simulink model "satelite01"  (Simulink 8.5)
settings: Solver=ode4  StartTime=0.0  StopTime=tfin  FixedStep=1/80
values from neighbouring files (symbols this model uses):
  A = [0 0 0.25 0.75 0 0;         0 0 0 0 2.52632 0;         0.75 0 0 0 0 0;         1 0 0 0 0 1;     0 1 0 0 0 0;     0 0 1 -1 0 0]    [Acoplado.m]    (also in insat03.m)
  B = [-0.25 0 0;     0 -0.842105 0;     0 0 0.75;     0 0 0;     0 0 0;     0 0 0]    [Acoplado.m]    (also in insat03.m = [-0.25 0 0;0 -0.842105 0;0 0 0.75)
  C = eye(6,6)    [Acoplado.m]    (also in insat03.m)
  D = zeros(6,3)    [Acoplado.m]    (also in insat03.m)
  ic = [0 0 0 0 0 0]    [Acoplado.m]    (also in insat03.m)
undefined symbols (not defined in the file or in its folder): K
libraries: simulink x1
settings Model: Creator=Vargas  LastModifiedBy=Admin
settings DataIOCC: SignalLoggingName=sigsOut
settings OptimizationCC: BlockReduction=off  BooleanDataType=off  InitFltsAndDblsToZero=on
settings DebuggingCC: SaveWithParameterizedLinksMsg=none  SignalResolutionControl=TryResolveAllWithWarning  MultiTaskDSMMsg=warning  MultiTaskCondExecSysMsg=none  FcnCallInpInsideContextMsg=UseLocalSettings  StrictBusMsg=None
settings HardwareCC: TargetUnknown=on

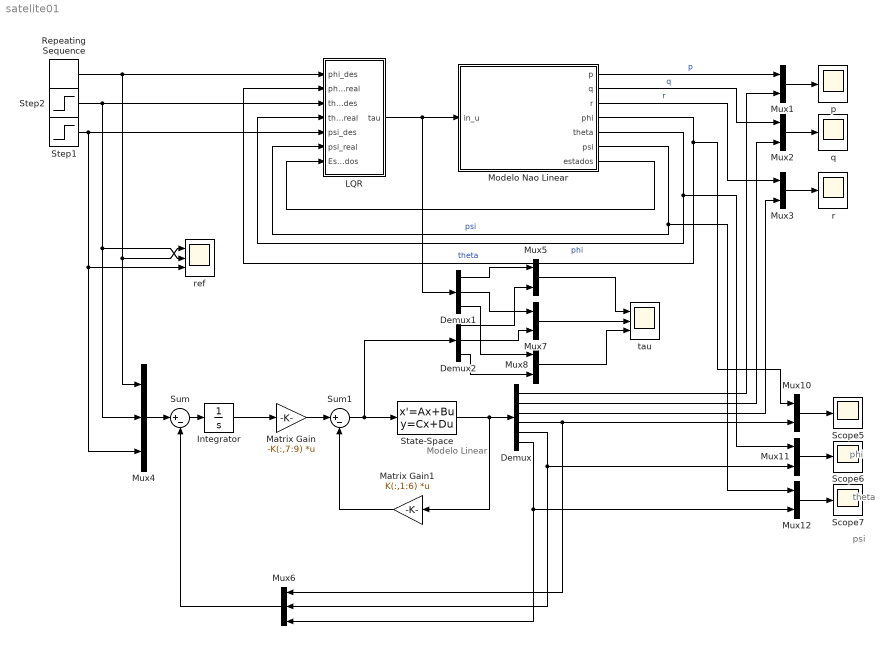
== system satelite01 ==
  note: phi
  note: theta
  note: psi
  note: Modelo Linear
  Demux : Demux  Outputs=6
  Demux1 : Demux  Outputs=3
  Demux2 : Demux  Outputs=3
  Integrator : Integrator
  LQR : Subsystem
  Matrix Gain : Gain  Gain=-K(:,7:9)  Multiplication=Matrix(K*u)  SaturateOnIntegerOverflow=on  OutDataTypeStr=Inherit: Same as input  ParamDataTypeStr=Inherit: Same as input
  Matrix Gain1 : Gain  Gain=K(:,1:6)  Multiplication=Matrix(K*u)  SaturateOnIntegerOverflow=on  OutDataTypeStr=Inherit: Same as input  ParamDataTypeStr=Inherit: Same as input
  Modelo Nao Linear : Subsystem
      mask Display: image(imread('Satelite3DOF_02.png'))
  Mux{1..3,5,7..8,10..12} (9 alike) : Mux  Inputs=2
  Mux4 : Mux  Inputs=3
  Mux6 : Mux  Inputs=3
  Repeating Sequence : simulink/Sources/Repeating Sequence  rep_seq_t=[0 5 15 30 40 50]  rep_seq_y="[0 0 0.5 0.5 0  0]"
  Scope5 : Scope
      settings: TimeRange=50  YMin=-1  YMax=1  SaveName=ScopeData06
  Scope6 : Scope
      settings: SaveName=ScopeData07
  Scope7 : Scope
      settings: SaveName=ScopeData08
  State-Space : StateSpace  A=A  B=B  C=C  D=D  X0=ic
  Step1 : Step  Time=0  After=0  SampleTime=0
  Step2 : Step  After=pi/4  SampleTime=0
  Sum : Sum  Inputs=|+-  SaturateOnIntegerOverflow=on
  Sum1 : Sum  Inputs=|+-  SaturateOnIntegerOverflow=on
  p : Scope
      settings: TickLabels=on  TimeRange=10  YMin=-0.8  YMax=0.8  SaveName=ScopeData03
  q : Scope
      settings: TickLabels=on  TimeRange=6  YMin=0.235  YMax=0.3  SaveName=ScopeData04
  r : Scope
      settings: TickLabels=on  TimeRange=10  YMin=0  YMax=600  SaveName=ScopeData05
  ref : Scope  NumInputPorts=3
      settings: TickLabels=on  TimeRange=50  YMin=-7000~-5~-5  YMax=6000~5~5  SaveName=ScopeData01
  tau : Scope  NumInputPorts=3
      settings: TickLabels=on  TimeRange=50  YMin=-7000~-5~-5  YMax=6000~5~5  SaveName=ScopeData02
  wires:
  Repeating Sequence/1 -> ref/1, Mux4/1, LQR/1(phi_des)
  Step2/1 -> ref/2, Mux4/2, LQR/3(theta_des)
  Step1/1 -> ref/3, Mux4/3, LQR/5(psi_des)
  Modelo Nao Linear/4(phi) -> Mux10/1, LQR/2(phi_real)  "theta"
  Modelo Nao Linear/5(theta) -> Mux11/1, LQR/4(theta_real)  "phi"
  Modelo Nao Linear/6(psi) -> Mux12/1, LQR/6(psi_real)  "psi"
  Modelo Nao Linear/7(estados) -> LQR/7(Estados)
  LQR/1(tau) -> Modelo Nao Linear/1(in_u), Demux1/1
  Modelo Nao Linear/3(r) -> Mux3/1  "r"
  Modelo Nao Linear/2(q) -> Mux2/1  "q"
  Modelo Nao Linear/1(p) -> Mux1/1  "p"
  Mux1/1 -> p/1
  Mux2/1 -> q/1
  Mux3/1 -> r/1
  State-Space/1 -> Demux/1, Matrix Gain1/1
  Sum1/1 -> State-Space/1, Demux2/1
  Matrix Gain/1 -> Sum1/1
  Integrator/1 -> Matrix Gain/1
  Sum/1 -> Integrator/1
  Matrix Gain1/1 -> Sum1/2
  Mux4/1 -> Sum/1
  Mux6/1 -> Sum/2
  Demux/5 -> Mux6/2, Mux11/2
  Demux/6 -> Mux6/3, Mux12/2
  Demux/1 -> Mux1/2
  Demux/3 -> Mux3/2
  Demux/4 -> Mux6/1, Mux10/2
  Mux10/1 -> Scope5/1
  Mux12/1 -> Scope7/1
  Mux11/1 -> Scope6/1
  Mux8/1 -> tau/3
  Mux5/1 -> tau/1
  Mux7/1 -> tau/2
  Demux/2 -> Mux2/2
  Demux1/1 -> Mux5/1
  Demux1/2 -> Mux7/1
  Demux1/3 -> Mux8/1
  Demux2/1 -> Mux5/2
  Demux2/2 -> Mux7/2
  Demux2/3 -> Mux8/2

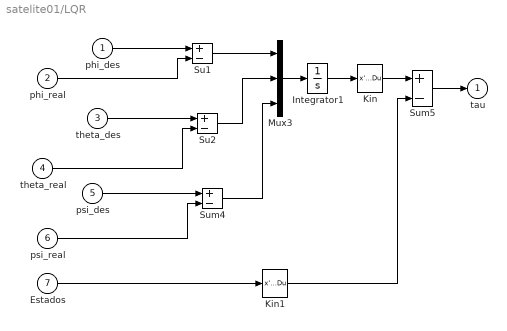
== system satelite01/LQR ==
  phi_des : Inport
  phi_real : Inport  Port=2
  theta_des : Inport  Port=3
  theta_real : Inport  Port=4
  psi_des : Inport  Port=5
  psi_real : Inport  Port=6
  Estados : Inport  Port=7
  Integrator1 : Integrator
  Kin : StateSpace  A=[]  B=[]  C=[]  D=K  X0=0  mask(Matrix Gain){K=-K(:,7:9)}
      mask prompts: K "Gain matrix:"
      mask help: Matrix Gain.
      mask Help: Multiplies input vector by entered matrix to produce output vector (y=Au).
      mask Display: disp('K')
  Kin1 : StateSpace  A=[]  B=[]  C=[]  D=K  X0=0  mask(Matrix Gain){K=K(:,1:6)}
      mask prompts: K "Gain matrix:"
      mask help: Matrix Gain.
      mask Help: Multiplies input vector by entered matrix to produce output vector (y=Au).
      mask Display: disp('K')
  Mux3 : Mux  Inputs=3
  Su1 : Sum  Inputs=+-  SaturateOnIntegerOverflow=on  InputSameDT=on  OutDataTypeStr=Inherit: Same as first input
  Su2 : Sum  Inputs=+-  SaturateOnIntegerOverflow=on  InputSameDT=on  OutDataTypeStr=Inherit: Same as first input
  Sum4 : Sum  Inputs=+-  SaturateOnIntegerOverflow=on  InputSameDT=on  OutDataTypeStr=Inherit: Same as first input
  Sum5 : Sum  Inputs=+-  SaturateOnIntegerOverflow=on  InputSameDT=on  OutDataTypeStr=Inherit: Same as first input
  tau : Outport
  wires:
  Su1/1 -> Mux3/1
  Su2/1 -> Mux3/2
  phi_real/1 -> Su1/2
  phi_des/1 -> Su1/1
  theta_des/1 -> Su2/1
  theta_real/1 -> Su2/2
  psi_des/1 -> Sum4/1
  psi_real/1 -> Sum4/2
  Kin/1 -> Sum5/1
  Sum5/1 -> tau/1
  Sum4/1 -> Mux3/3
  Mux3/1 -> Integrator1/1
  Integrator1/1 -> Kin/1
  Estados/1 -> Kin1/1
  Kin1/1 -> Sum5/2

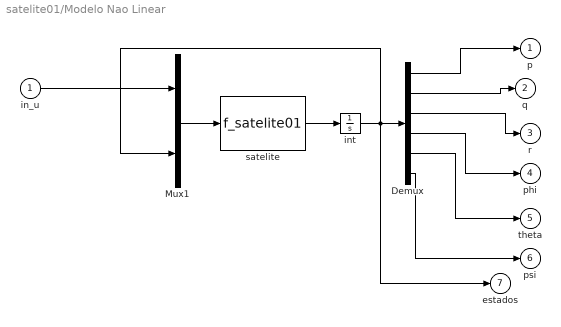
== system satelite01/Modelo Nao Linear ==
  in_u : Inport
  Demux : Demux  Outputs=6
  Mux1 : Mux  Inputs=2
  int : Integrator  InitialCondition=ic
  satelite : S-Function  FunctionName=f_satelite01  Parameters=o
  p : Outport
  q : Outport  Port=2
  r : Outport  Port=3
  phi : Outport  Port=4
  theta : Outport  Port=5
  psi : Outport  Port=6
  estados : Outport  Port=7
  wires:
  Mux1/1 -> satelite/1
  in_u/1 -> Mux1/1
  satelite/1 -> int/1
  int/1 -> Mux1/2, Demux/1, estados/1
  Demux/1 -> p/1
  Demux/2 -> q/1
  Demux/3 -> r/1
  Demux/4 -> phi/1
  Demux/5 -> theta/1
  Demux/6 -> psi/1
